simulink model "debug"  (R2024a)
settings: Solver=VariableStepAuto  StartTime=0.0  StopTime=4  RelTol=1e-3
model workspace (MAT data in the model file):
  Frequency_175 = 0
  TargetFrequency_175 = 2100000000
  uniqueStringPll_175 = '53_5733'
undefined symbols (not defined in the file): DiscIntNeverNeededParam
libraries: simulink x4, mcbcontrolslib x1, slpidlib x1
settings Model: Creator=wsl  LastModifiedBy=wsl

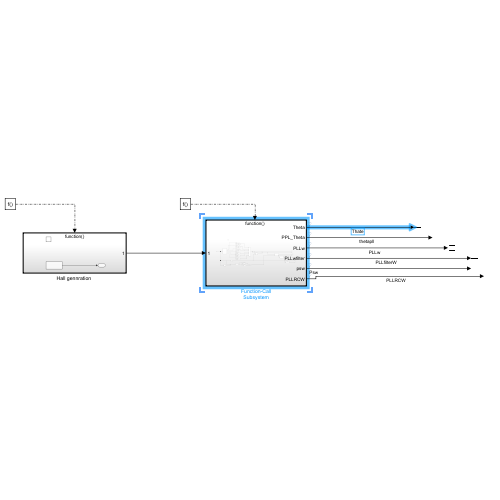
[thumbnail: Simulink's stored preview of the top-level diagram]
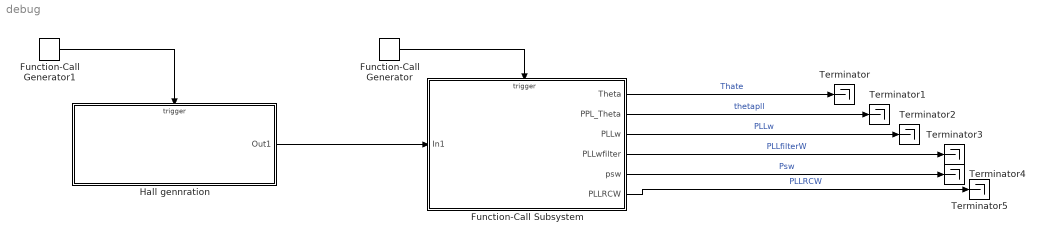
== system debug ==
  Function-Call Generator : simulink/Ports & Subsystems/Function-Call Generator  sample_time=1e-4  numberOfIterations=1  DisallowWideOutput=off
  Function-Call Generator1 : simulink/Ports & Subsystems/Function-Call Generator  sample_time=1/48  numberOfIterations=1  DisallowWideOutput=off
  Function-Call Subsystem : Subsystem  TreatAsAtomicUnit=on
  "Hall gennration " : Subsystem  TreatAsAtomicUnit=on
  Terminator{,1..5} (6 alike) : Terminator
  wires:
  Function-Call Generator/1 -> Function-Call Subsystem/Trigger
  Function-Call Generator1/1 -> "Hall gennration "/Trigger
  "Hall gennration "/1(Out1) -> Function-Call Subsystem/1(In1)
  Function-Call Subsystem/1(Theta) -> Terminator/1  "Thate"
  Function-Call Subsystem/2(PPL_Theta) -> Terminator1/1  "thetapll"
  Function-Call Subsystem/3(PLLw) -> Terminator2/1  "PLLw"
  Function-Call Subsystem/4(PLLwfilter) -> Terminator3/1  "PLLfilterW"
  Function-Call Subsystem/6(PLLRCW) -> Terminator5/1  "PLLRCW"
  Function-Call Subsystem/5(psw) -> Terminator4/1  "Psw"

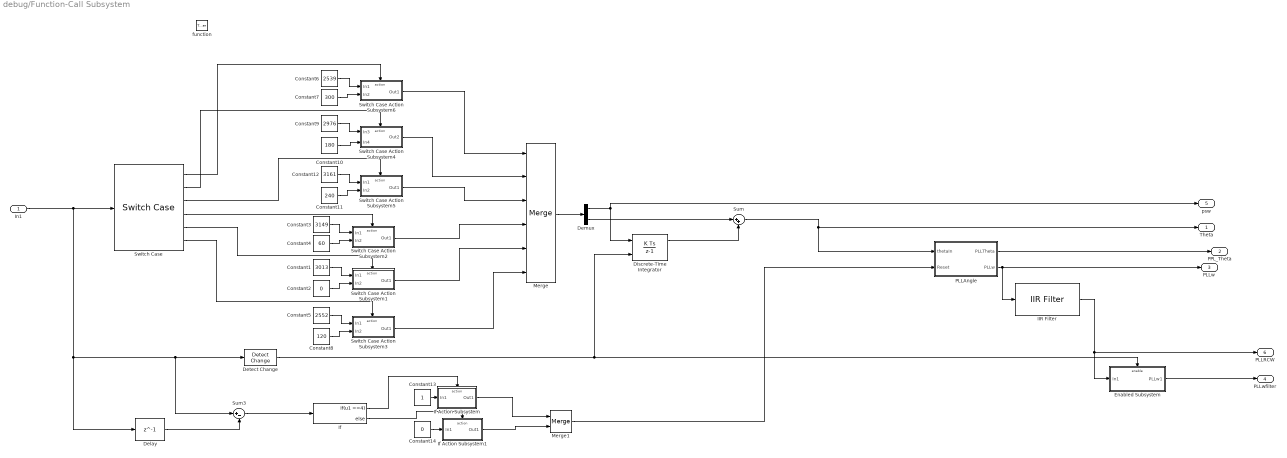
== system debug/Function-Call Subsystem ==
  In1 : Inport
  function : TriggerPort  TriggerType=function-call  VariantControl=(inherit)
  Constant1 : Constant  Value=3013
  Constant10 : Constant  Value=180
  Constant11 : Constant  Value=240
  Constant12 : Constant  Value=3161
  Constant13 : Constant  OutDataTypeStr=boolean
  Constant14 : Constant  Value=0  OutDataTypeStr=boolean
  Constant2 : Constant  Value=0
  Constant3 : Constant  Value=3149
  Constant4 : Constant  Value=60
  Constant5 : Constant  Value=2552
  Constant6 : Constant  Value=2539
  Constant7 : Constant  Value=300
  Constant8 : Constant  Value=120
  Constant9 : Constant  Value=2976
  Delay : Delay  DelayLength=1  InitialCondition=0  UseCircularBuffer=on
  Demux : Demux  Outputs=2
  Detect Change : simulink/Logic and Bit Operations/Detect Change  vinit=0  OutDataTypeStr=boolean
  Discrete-Time Integrator : DiscreteIntegrator  ExternalReset=rising  SampleTime=-1  LimitOutput=on  UpperSaturationLimit=60  LowerSaturationLimit=-60  ShowSaturationPort=on  ICPrevOutput=DiscIntNeverNeededParam  ICPrevScaledInput=DiscIntNeverNeededParam
  Enabled Subsystem : Subsystem  TreatAsAtomicUnit=on
  IIR Filter : mcbcontrolslib/IIR Filter  VariantControl=Low Pass Filter  VariantSelect=Low-pass  FilterConstantInputType=Specify via dialog  Filter_constant=0.01  advancedSettings=on  Ts=1e-4  cutOff_freq=16.0763
      settings: LibrarySourceBlock=mcbhdllib/Signal Management/IIR Filter
  If : If  IfExpression=u1 ==4
  If Action Subsystem : Subsystem  TreatAsAtomicUnit=on
  If Action Subsystem1 : Subsystem  TreatAsAtomicUnit=on
  Merge : Merge  Inputs=6
  Merge1 : Merge
  PLLAngle : Subsystem
  Sum : Sum  Inputs=|++
  Sum3 : Sum  Inputs=|+-
  Switch Case : SwitchCase  CaseConditions={1,2,3,4,5,6}  ShowDefaultCase=off
  Switch Case Action Subsystem1 : Subsystem  TreatAsAtomicUnit=on
  Switch Case Action Subsystem2 : Subsystem  TreatAsAtomicUnit=on
  Switch Case Action Subsystem3 : Subsystem  TreatAsAtomicUnit=on
  Switch Case Action Subsystem4 : Subsystem  TreatAsAtomicUnit=on
  Switch Case Action Subsystem5 : Subsystem  TreatAsAtomicUnit=on
  Switch Case Action Subsystem6 : Subsystem  TreatAsAtomicUnit=on
  Theta : Outport
  PPL_Theta : Outport  Port=2
  PLLw : Outport  Port=3
  PLLwfilter : Outport  Port=4
  psw : Outport  Port=5
  PLLRCW : Outport  Port=6
  wires:
  In1/1 -> Delay/1, Sum3/1, Detect Change/1, Switch Case/1
  Switch Case/1 -> Switch Case Action Subsystem6/Action
  Constant6/1 -> Switch Case Action Subsystem6/1(In1)
  Constant7/1 -> Switch Case Action Subsystem6/2(In2)
  Constant2/1 -> Switch Case Action Subsystem1/2(In2)
  Constant1/1 -> Switch Case Action Subsystem1/1(In1)
  Switch Case/5 -> Switch Case Action Subsystem1/Action
  Constant4/1 -> Switch Case Action Subsystem2/2(In2)
  Constant3/1 -> Switch Case Action Subsystem2/1(In1)
  Switch Case/4 -> Switch Case Action Subsystem2/Action
  Constant8/1 -> Switch Case Action Subsystem3/2(In2)
  Constant5/1 -> Switch Case Action Subsystem3/1(In1)
  Switch Case/6 -> Switch Case Action Subsystem3/Action
  Constant9/1 -> Switch Case Action Subsystem4/1(In3)
  Constant10/1 -> Switch Case Action Subsystem4/2(In4)
  Switch Case/2 -> Switch Case Action Subsystem4/Action
  Constant12/1 -> Switch Case Action Subsystem5/1(In1)
  Constant11/1 -> Switch Case Action Subsystem5/2(In2)
  Switch Case/3 -> Switch Case Action Subsystem5/Action
  Switch Case Action Subsystem6/1(Out1) -> Merge/1
  Switch Case Action Subsystem4/1(Out2) -> Merge/2
  Switch Case Action Subsystem5/1(Out1) -> Merge/3
  Switch Case Action Subsystem2/1(Out1) -> Merge/4
  Switch Case Action Subsystem1/1(Out1) -> Merge/5
  Switch Case Action Subsystem3/1(Out1) -> Merge/6
  Merge/1 -> Demux/1
  Demux/1 -> Discrete-Time Integrator/1, psw/1
  Discrete-Time Integrator/1 -> Sum/2
  Demux/2 -> Sum/1
  Detect Change/1 -> Enabled Subsystem/Enable, Discrete-Time Integrator/2
  Sum/1 -> PLLAngle/1(thetaIn), Theta/1
  Delay/1 -> Sum3/2
  Sum3/1 -> If/1
  If/1 -> If Action Subsystem/Action
  Constant13/1 -> If Action Subsystem/1(In1)
  If/2 -> If Action Subsystem1/Action
  Constant14/1 -> If Action Subsystem1/1(In1)
  If Action Subsystem/1(Out1) -> Merge1/1
  If Action Subsystem1/1(Out1) -> Merge1/2
  IIR Filter/1 -> PLLRCW/1, Enabled Subsystem/1(In1)
  Enabled Subsystem/1(PLLw1) -> PLLwfilter/1
  PLLAngle/2(PLLw) -> PLLw/1, IIR Filter/1
  Merge1/1 -> PLLAngle/2(Reset)
  PLLAngle/1(PLLTheta) -> PPL_Theta/1

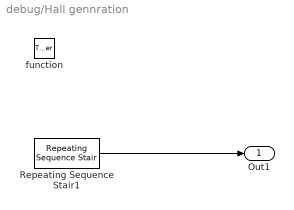
== system debug/Hall gennration  ==
  function : TriggerPort  TriggerType=function-call  VariantControl=(inherit)
  Repeating Sequence Stair1 : simulink/Sources/Repeating Sequence Stair  OutValues=[1 5 4 6 2 3].'  tsamp=-1  OutMin=[]  OutMax=[]  OutDataTypeStr=double  OutputDataTypeScalingMode=double  OutDataType=fixdt(0,8)  ConRadixGroup=Best Precision: Vector-wise  OutScaling=2^-12
  Out1 : Outport
  wires:
  Repeating Sequence Stair1/1 -> Out1/1

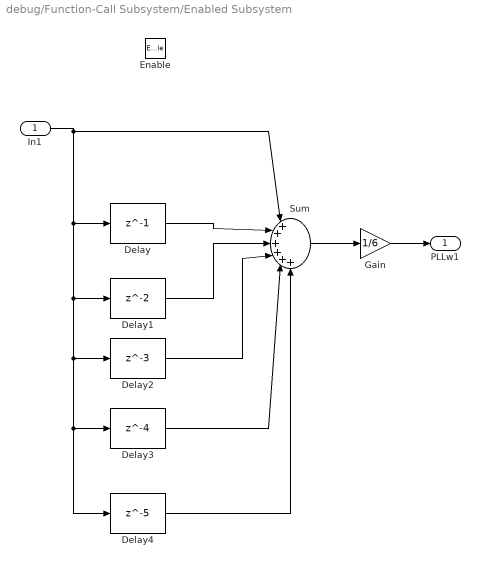
== system debug/Function-Call Subsystem/Enabled Subsystem ==
  In1 : Inport
  Enable : EnablePort
  Delay : Delay  DelayLength=1  InitialCondition=0  UseCircularBuffer=on
  Delay1 : Delay  InitialCondition=0  UseCircularBuffer=on
  Delay2 : Delay  DelayLength=3  InitialCondition=0  UseCircularBuffer=on
  Delay3 : Delay  DelayLength=4  InitialCondition=0  UseCircularBuffer=on
  Delay4 : Delay  DelayLength=5  InitialCondition=0  UseCircularBuffer=on
  Gain : Gain  Gain=1/6
  Sum : Sum  Inputs=|++++++
  PLLw1 : Outport
  wires:
  In1/1 -> Delay4/1, Delay3/1, Delay2/1, Delay1/1, Delay/1, Sum/1
  Delay/1 -> Sum/2
  Delay1/1 -> Sum/3
  Sum/1 -> Gain/1
  Gain/1 -> PLLw1/1
  Delay2/1 -> Sum/4
  Delay3/1 -> Sum/5
  Delay4/1 -> Sum/6

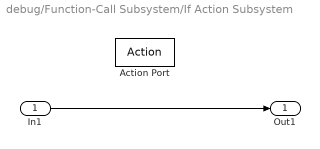
== system debug/Function-Call Subsystem/If Action Subsystem ==
  In1 : Inport
  Action Port : ActionPort  ActionPortLabel=if(u1 ==4)
  Out1 : Outport
  wires:
  In1/1 -> Out1/1

== system debug/Function-Call Subsystem/If Action Subsystem1 ==
  In1 : Inport
  Action Port : ActionPort  ActionPortLabel=else
  Out1 : Outport
  wires:
  In1/1 -> Out1/1

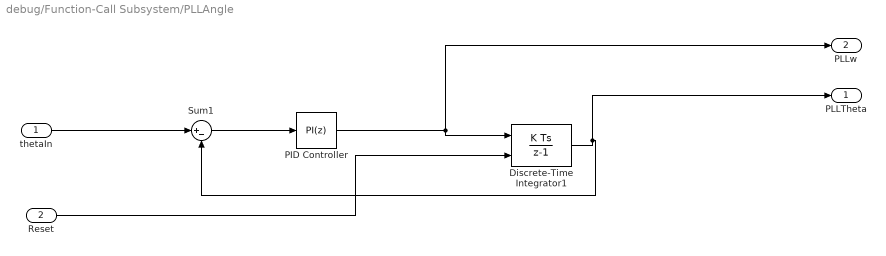
== system debug/Function-Call Subsystem/PLLAngle ==
  thetaIn : Inport
  Reset : Inport  Port=2
  Discrete-Time Integrator1 : DiscreteIntegrator  ExternalReset=rising  SampleTime=-1  LimitOutput=on  UpperSaturationLimit=360  LowerSaturationLimit=0  IgnoreLimit=on  ICPrevOutput=DiscIntNeverNeededParam  ICPrevScaledInput=DiscIntNeverNeededParam
  PID Controller : slpidlib/PID Controller  Controller=PI  Form=Parallel  TimeDomain=Discrete-time  UseExternalTs=off  SampleTime=-1  IntegratorMethod=Forward Euler  FilterMethod=Forward Euler  ControllerParametersSource=internal  P=530  I=0.28  UseKiTs=off  D=0  UseExternalDerivativeSource=off  N=100  UseFilter=on  TunerSelectOption=Transfer Function Based (PID Tuner App)  InitialConditionSource=internal  InitialConditionForIntegrator=0  InitialConditionForFilter=0  DifferentiatorICPrevScaledInput=0  ExternalReset=none  TrackingMode=off  Kt=1  LimitOutput=off  SatLimitsSource=internal  UpperSaturationLimit=inf  LowerSaturationLimit=-inf  LinearizeAsGain=on  AntiWindupMode=none  Kb=1  LimitIntegrator=off  UpperIntegratorSaturationLimit=inf  LowerIntegratorSaturationLimit=-inf  POutMin=[]  POutMax=[]  IOutMin=[]  IOutMax=[]  DOutMin=[]  DOutMax=[]  NOutMin=[]  NOutMax=[]  SumOutMin=[]  SumOutMax=[]  SaturationOutMin=[]  SaturationOutMax=[]  PParamMin=[]  PParamMax=[]  IParamMin=[]  IParamMax=[]  DParamMin=[]  DParamMax=[]  NParamMin=[]  NParamMax=[]  KbParamMin=[]  KbParamMax=[]  KtParamMin=[]  KtParamMax=[]  KbOutMin=[]  KbOutMax=[]  KtOutMin=[]  KtOutMax=[]  IntegratorOutMin=[]  IntegratorOutMax=[]  FilterOutMin=[]  FilterOutMax=[]  SumI1OutMin=[]  SumI1OutMax=[]  SumI2OutMin=[]  SumI2OutMax=[]  SumI3OutMin=[]  SumI3OutMax=[]  SumI4OutMin=[]  SumI4OutMax=[]  SumDOutMin=[]  SumDOutMax=[]  DifferentiatorOutMin=[]  DifferentiatorOutMax=[]  FilterDiffOutCoefMin=[]  FilterDiffOutCoefMax=[]  ReciprocalOutMin=[]  ReciprocalOutMax=[]  SumDenOutMin=[]  SumDenOutMax=[]  SumNumOutMin=[]  SumNumOutMax=[]  DivideOutMin=[]  DivideOutMax=[]  UdiffTsProdOutMin=[]  UdiffTsProdOutMax=[]  NTsProdOutMin=[]  NTsProdOutMax=[]  UintegralTsProdOutMin=[]  UintegralTsProdOutMax=[]  UngainTsProdOutMin=[]  UngainTsProdOutMax=[]  ClampingZeroOutDataTypeStr=Inherit: Inherit via back propagation  ClampingZeroOutMin=[]  ClampingZeroOutMax=[]  FilterDenConstantOutDataTypeStr=Inherit: Inherit via back propagation  FilterDenConstantOutMin=[]  FilterDenConstantOutMax=[]  PCopyOutDataTypeStr=Inherit: Inherit via back propagation  PCopyOutMin=[]  PCopyOutMax=[]  NCopyOutDataTypeStr=Inherit: Inherit via back propagation  NCopyOutMin=[]  NCopyOutMax=[]  IntegratorContinuousStateAttributes=''  IntegratorStateMustResolveToSignalObject=off  IntegratorRTWStateStorageClass=Auto  FilterContinuousStateAttributes=''  FilterStateMustResolveToSignalObject=off  FilterRTWStateStorageClass=Auto  ParallelPVariant=InternalParameters  IdealPVariant=Disabled  IVariant=InternalParameters  DVariant=Disabled  IntegratorVariant=Discrete  SatVariant=Disabled  AWVariant=Passthrough  PCopyVariant=Disabled  TRVariant=Disabled  FdbkBlocksVariant=Forward  IdealPFdbkVariant=Disabled  SatFdbkVariant=Disabled  DerivativeFilterVariant=Disabled  NVariant=Disabled  NCopyVariant=Disabled_SignalSpec  FilterICVariant=Disabled  IntegratorICVariant=InternalICs  ExternalResetVariant=Disabled  TRSumVariant=Passthrough  SumFdbkVariant=Disabled  SumVariant=Sum_PI  TsampFilterVariant=InternalTs  TsampNgainVariant=Passthrough  TsampIntegralVariant=Disabled_SignalSpec  ExternalSaturationOutDataTypeStr=Inherit: Same as second input  DerivativeSourceVariant=Disabled
  Sum1 : Sum  Inputs=|+-
  PLLTheta : Outport
  PLLw : Outport  Port=2
  wires:
  Sum1/1 -> PID Controller/1
  Discrete-Time Integrator1/1 -> PLLTheta/1, Sum1/2
  thetaIn/1 -> Sum1/1
  PID Controller/1 -> PLLw/1, Discrete-Time Integrator1/1
  Reset/1 -> Discrete-Time Integrator1/2

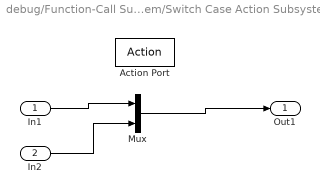
== system debug/Function-Call Subsystem/Switch Case Action Subsystem1 ==
  In1 : Inport
  In2 : Inport  Port=2
  Action Port : ActionPort  ActionPortLabel=case [ 5 ]:
  Mux : Mux  Inputs=2
  Out1 : Outport
  wires:
  In1/1 -> Mux/1
  In2/1 -> Mux/2
  Mux/1 -> Out1/1

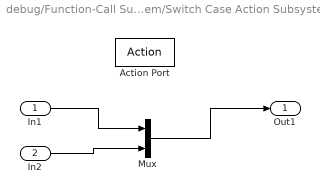
== system debug/Function-Call Subsystem/Switch Case Action Subsystem2 ==
  In1 : Inport
  In2 : Inport  Port=2
  Action Port : ActionPort  ActionPortLabel=case [ 4 ]:
  Mux : Mux  Inputs=2
  Out1 : Outport
  wires:
  In1/1 -> Mux/1
  In2/1 -> Mux/2
  Mux/1 -> Out1/1

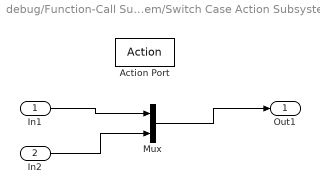
== system debug/Function-Call Subsystem/Switch Case Action Subsystem3 ==
  In1 : Inport
  In2 : Inport  Port=2
  Action Port : ActionPort  ActionPortLabel=case [ 6 ]:
  Mux : Mux  Inputs=2
  Out1 : Outport
  wires:
  In1/1 -> Mux/1
  In2/1 -> Mux/2
  Mux/1 -> Out1/1

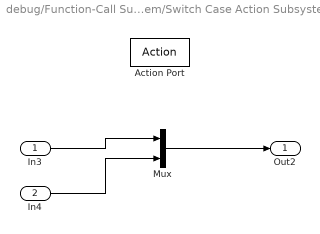
== system debug/Function-Call Subsystem/Switch Case Action Subsystem4 ==
  In3 : Inport
  In4 : Inport  Port=2
  Action Port : ActionPort  ActionPortLabel=case [ 2 ]:
  Mux : Mux  Inputs=2
  Out2 : Outport
  wires:
  Mux/1 -> Out2/1
  In3/1 -> Mux/1
  In4/1 -> Mux/2

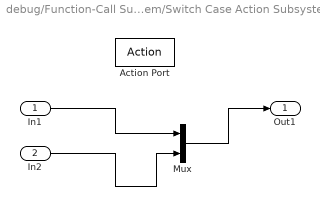
== system debug/Function-Call Subsystem/Switch Case Action Subsystem5 ==
  In1 : Inport
  In2 : Inport  Port=2
  Action Port : ActionPort  ActionPortLabel=case [ 3 ]:
  Mux : Mux  Inputs=2
  Out1 : Outport
  wires:
  In1/1 -> Mux/1
  In2/1 -> Mux/2
  Mux/1 -> Out1/1

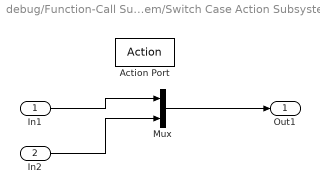
== system debug/Function-Call Subsystem/Switch Case Action Subsystem6 ==
  In1 : Inport
  In2 : Inport  Port=2
  Action Port : ActionPort  ActionPortLabel=case [ 1 ]:
  Mux : Mux  Inputs=2
  Out1 : Outport
  wires:
  Mux/1 -> Out1/1
  In1/1 -> Mux/1
  In2/1 -> Mux/2
